simulink model "Short_Circuit_Tests_of_Single_Phase_Transformer"  (R2025a)
settings: Solver=ode23tb  StartTime=0.0  StopTime=5  MaxStep=1e-4  RelTol=1e-3
libraries: spsRMSLib x2, spsCurrentMeasurementLib x1, spsLinearTransformerLib x1, spsPowerLib x1, spsVoltageMeasurementLib x1, spsACVoltageSourceLib x1, sps_lib x1
settings Model: Creator=Jawad  LastModifiedBy=Jawad

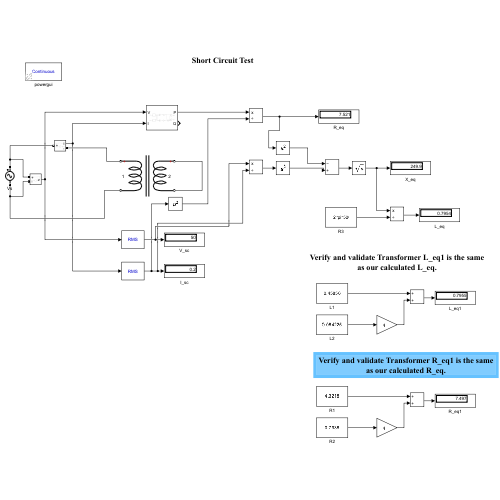
[thumbnail: Simulink's stored preview of the top-level diagram]
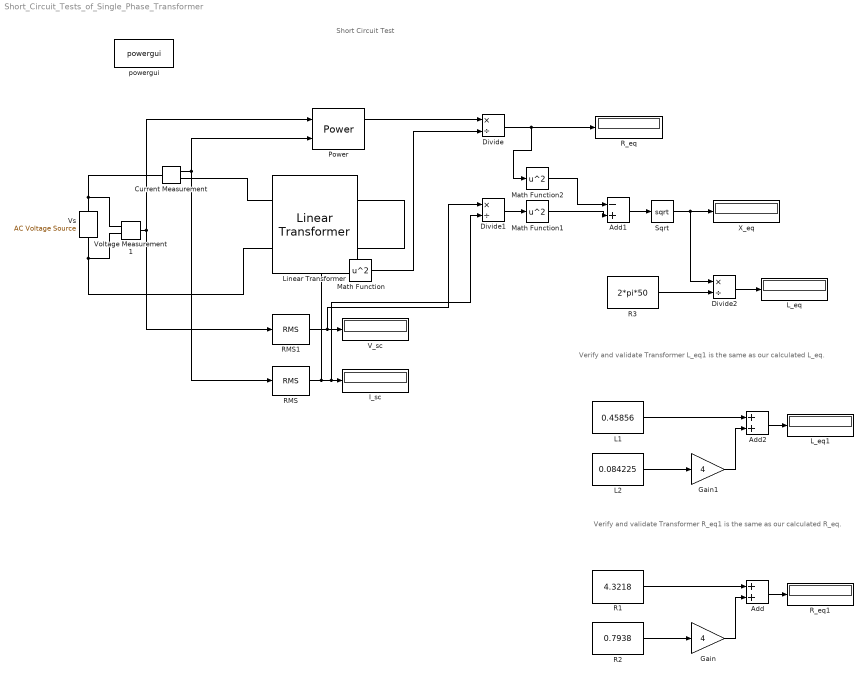
== system Short_Circuit_Tests_of_Single_Phase_Transformer ==
  note: Verify and validate Transformer R_eq1 is the same as our calculated R_eq.
  note: Short Circuit Test
  note: Verify and validate Transformer L_eq1 is the same as our calculated L_eq.
  Add : Sum
  Add1 : Sum  Inputs=-+
  Add2 : Sum
  Current Measurement : spsCurrentMeasurementLib/Current Measurement  PhasorSimulation=off  OutputType=Complex  PSBequivalent=0
  Divide : Product  Inputs=*/
  Divide1 : Product  Inputs=*/
  Divide2 : Product  Inputs=*/
  Gain : Gain  Gain=4
  Gain1 : Gain  Gain=4
  I_sc : Display
  L1 : Constant  Value=0.45856
  L2 : Constant  Value=0.084225
  L_eq : Display
  L_eq1 : Display
  Linear Transformer : spsLinearTransformerLib/Linear Transformer  UNITS=SI  NominalPower=[ 2000 50 ]  winding1=[220 4.3218 0.45856]  winding2=[110 0.7938 0.084225]  ThreeWindings=off  winding3=[3.15e+05 0.7938 0.084225]  RmLm=[1.0804e+06 2866]  Measurements=None  DataType=on
  Math Function : Math  Operator=square
  Math Function1 : Math  Operator=square
  Math Function2 : Math  Operator=square
  Power : spsPowerLib/Power  Freq=50  Vinit=[1, 0]  Iinit=[1, 0]  Ts=0
  R1 : Constant  Value=4.3218
  R2 : Constant  Value=0.7938
  R3 : Constant  Value=2*pi*50
  RMS : spsRMSLib/RMS  TrueRMS=off  Freq=50  RMSInit=0  Ts=0
  RMS1 : spsRMSLib/RMS  TrueRMS=off  Freq=50  RMSInit=0  Ts=0
  R_eq : Display
  R_eq1 : Display
  Sqrt : Sqrt
  V_sc : Display
  Voltage Measurement1 : spsVoltageMeasurementLib/Voltage Measurement  PhasorSimulation=off  OutputType=Complex  PSBequivalent=0
  Vs : spsACVoltageSourceLib/AC Voltage Source  Amplitude=50*sqrt(2)  Phase=0  Frequency=50  SampleTime=0  Measurements=None  BusType=swing  Pref=10e3  Qref=0  Qmin=-inf  Qmax=+inf
  X_eq : Display
  powergui : sps_lib/powergui  Priority=1  SimulationMode=Continuous  SampleTime=50e-6  frequency=60  Iterations=50  frequencyindice=50  Pbase=100e6  ErrMax=1e-4  UnitsV=kV  UnitsW=MW  buscounter=0  FunctionMessages=off  echomessages=off  EnableUseOfTLC=off  CurrentSourceSwitches=off  DisableSnubberDevices=off  DisableRonSwitches=off  DisableVfSwitches=off  DisplayEquations=off  AutomaticDiscreteSolvers=off  SolverType=Tustin/Backward Euler (TBE)  Interpol=off  ExternalGateDelay=off  methode=off  Ts=100  x0status=blocks  SPID=on  SwTol=0  HookPort=off  NonlinearTolerance=1e-4  nMaxIteration=100  ContinueOnMaxIteration=off  RestoreLinks=warning  ResistiveCurrentMeasurement=off  Frange=[0:2:500]  Ylog=off  Xlog=on  ShowGrid=off  save=off  variable=ZData  structure=0  ZoomFFT=off  StartTime=0.0  cycles=1  DisplayStyle=1  fundamental=60  FreqAxis=off  MaxFrequency=1000  frequencyindicesteady=1  RmsSteady=1  display=off
  wires:
  Current Measurement/1 -> RMS/1, Power/2
  RMS1/1 -> Divide1/1, V_sc/1
  Voltage Measurement1/1 -> RMS1/1, Power/1
  RMS/1 -> Divide1/2, I_sc/1, Math Function/1
  Power/1 -> Divide/1
  Math Function/1 -> Divide/2
  Divide/1 -> Math Function2/1, R_eq/1
  R2/1 -> Gain/1
  R1/1 -> Add/1
  Gain/1 -> Add/2
  Add/1 -> R_eq1/1
  Divide1/1 -> Math Function1/1
  Math Function2/1 -> Add1/1
  Math Function1/1 -> Add1/2
  Add1/1 -> Sqrt/1
  Sqrt/1 -> Divide2/1, X_eq/1
  R3/1 -> Divide2/2
  Divide2/1 -> L_eq/1
  Add2/1 -> L_eq1/1
  L1/1 -> Add2/1
  Gain1/1 -> Add2/2
  L2/1 -> Gain1/1
  connections:
  Vs/LConn1 -- Voltage Measurement1/LConn2 -- Linear Transformer/LConn2
  Vs/RConn1 -- Current Measurement/LConn1 -- Voltage Measurement1/LConn1
  Current Measurement/RConn1 -- Linear Transformer/LConn1
  Linear Transformer/RConn1 -- Linear Transformer/RConn2
